simulink model "SPWM_3ph_VSI"  (R2022b)
settings: Solver=FixedStepAuto  StartTime=0.0  StopTime=0.5  RelTol=1e-3
libraries: spsIGBTDiodeLib x6, spsSeriesRLCBranchLib x3, spsDCVoltageSourceLib x2, spsVoltageMeasurementLib x2, spsGroundLib x1, spsTriangleGeneratorLib x1, spspowerguiLib x1
settings Model: Creator=jack  LastModifiedBy=jack

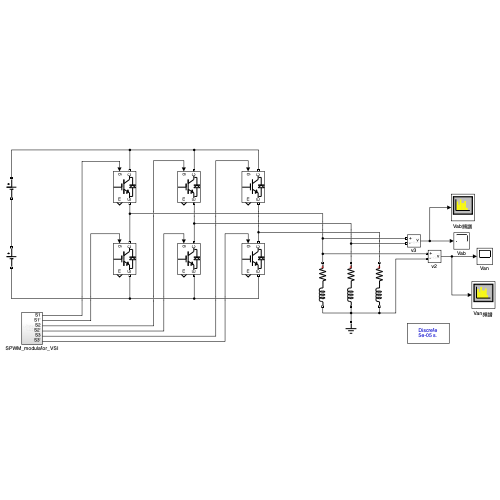
[thumbnail: Simulink's stored preview of the top-level diagram]
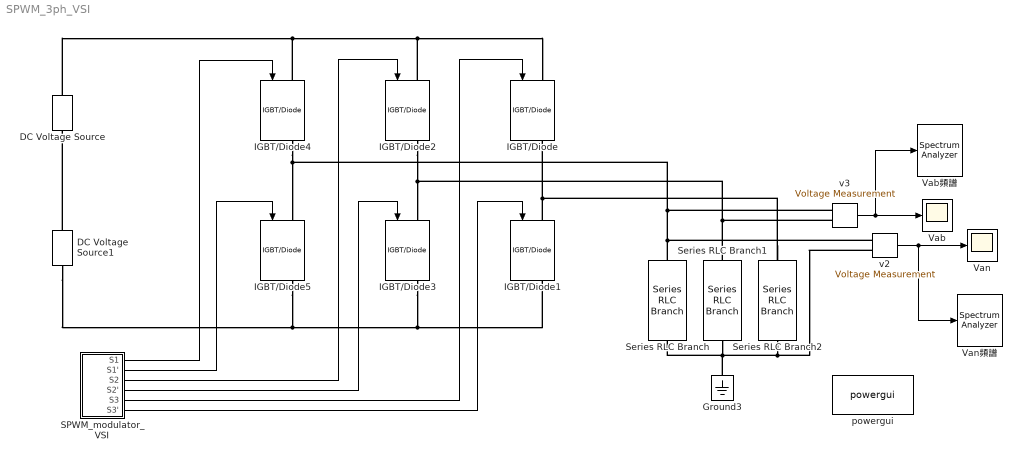
== system SPWM_3ph_VSI ==
  DC Voltage Source : spsDCVoltageSourceLib/DC Voltage Source  Amplitude=100  Measurements=None
  DC Voltage Source1 : spsDCVoltageSourceLib/DC Voltage Source  Amplitude=100  Measurements=None
  Ground3 : spsGroundLib/Ground  LConnTagsString=a
  IGBT/Diode{,1..5} (6 alike) : spsIGBTDiodeLib/IGBT//Diode  Ron=1e-3  Rs=1e5  Cs=inf  Measurements=on
  SPWM_modulator_VSI : Subsystem
  Series RLC Branch : spsSeriesRLCBranchLib/Series RLC Branch  LConnTagsString=__new0  RConnTagsString=__new0  BranchType=RL  Resistance=5  Inductance=150e-3  SetiL0=off  InitialCurrent=0  Capacitance=0  Setx0=off  InitialVoltage=0  Measurements=None
  Series RLC Branch1 : spsSeriesRLCBranchLib/Series RLC Branch  LConnTagsString=__new0  RConnTagsString=__new0  BranchType=RL  Resistance=5  Inductance=150e-3  SetiL0=off  InitialCurrent=0  Capacitance=0  Setx0=off  InitialVoltage=0  Measurements=None
  Series RLC Branch2 : spsSeriesRLCBranchLib/Series RLC Branch  LConnTagsString=__new0  RConnTagsString=__new0  BranchType=RL  Resistance=5  Inductance=150e-3  SetiL0=off  InitialCurrent=0  Capacitance=0  Setx0=off  InitialVoltage=0  Measurements=None
  Vab : Scope
  Vab頻譜 : SpectrumAnalyzer
  Van : Scope
  Van頻譜 : SpectrumAnalyzer
  powergui : spspowerguiLib/powergui  Priority=1  SimulationMode=Discrete  SampleTime=50e-6  frequency=60  Iterations=50  frequencyindice=0  Pbase=100e6  ErrMax=1e-4  UnitsV=kV  UnitsW=MW  buscounter=0  FunctionMessages=off  echomessages=off  EnableUseOfTLC=off  CurrentSourceSwitches=off  DisableSnubberDevices=off  DisableRonSwitches=off  DisableVfSwitches=off  DisplayEquations=off  AutomaticDiscreteSolvers=off  SolverType=Tustin/Backward Euler (TBE)  Interpol=off  ExternalGateDelay=off  methode=off  Ts=100  x0status=blocks  SPID=on  SwTol=0  HookPort=off  NonlinearTolerance=1e-4  nMaxIteration=100  ContinueOnMaxIteration=off  RestoreLinks=warning  ResistiveCurrentMeasurement=off  Frange=[0:2:500]  Ylog=off  Xlog=on  ShowGrid=off  save=off  variable=ZData  structure=0  ZoomFFT=off  StartTime=0.0  cycles=1  DisplayStyle=1  fundamental=60  FreqAxis=off  MaxFrequency=1000  frequencyindicesteady=1  RmsSteady=1  display=off
  v2 : spsVoltageMeasurementLib/Voltage Measurement  PhasorSimulation=off  OutputType=Complex  PSBequivalent=0
  v3 : spsVoltageMeasurementLib/Voltage Measurement  PhasorSimulation=off  OutputType=Complex  PSBequivalent=0
  wires:
  v2/1 -> Van頻譜/1, Van/1
  v3/1 -> Vab頻譜/1, Vab/1
  SPWM_modulator_VSI/1(S1) -> IGBT/Diode4/1
  SPWM_modulator_VSI/2(S1') -> IGBT/Diode5/1
  SPWM_modulator_VSI/3(S2) -> IGBT/Diode2/1
  SPWM_modulator_VSI/4(S2') -> IGBT/Diode3/1
  SPWM_modulator_VSI/5(S3) -> IGBT/Diode/1
  SPWM_modulator_VSI/6(S3') -> IGBT/Diode1/1
  connections:
  IGBT/Diode1/LConn1 -- IGBT/Diode/RConn1 -- Series RLC Branch2/LConn1
  IGBT/Diode1/RConn1 -- DC Voltage Source1/LConn1 -- IGBT/Diode5/RConn1 -- IGBT/Diode3/RConn1
  DC Voltage Source/RConn1 -- IGBT/Diode4/LConn1 -- IGBT/Diode2/LConn1 -- IGBT/Diode/LConn1
  IGBT/Diode2/RConn1 -- Series RLC Branch1/LConn1 -- v3/LConn2 -- IGBT/Diode3/LConn1
  IGBT/Diode4/RConn1 -- v3/LConn1 -- v2/LConn1 -- Series RLC Branch/LConn1 -- IGBT/Diode5/LConn1
  DC Voltage Source1/RConn1 -- DC Voltage Source/LConn1
  Series RLC Branch1/RConn1 -- v2/LConn2 -- Series RLC Branch2/RConn1 -- Series RLC Branch/RConn1 -- Ground3/LConn1

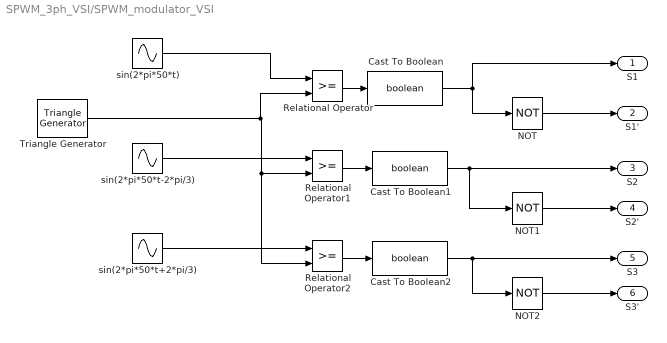
== system SPWM_3ph_VSI/SPWM_modulator_VSI ==
  Cast To Boolean : DataTypeConversion  OutDataTypeStr=boolean  SaturateOnIntegerOverflow=off  RndMeth=Floor
  Cast To Boolean1 : DataTypeConversion  OutDataTypeStr=boolean  SaturateOnIntegerOverflow=off  RndMeth=Floor
  Cast To Boolean2 : DataTypeConversion  OutDataTypeStr=boolean  SaturateOnIntegerOverflow=off  RndMeth=Floor
  NOT : Logic  Operator=NOT  IconShape=distinctive  AllPortsSameDT=off  OutDataTypeStr=boolean
  NOT1 : Logic  Operator=NOT  IconShape=distinctive  AllPortsSameDT=off  OutDataTypeStr=boolean
  NOT2 : Logic  Operator=NOT  IconShape=distinctive  AllPortsSameDT=off  OutDataTypeStr=boolean
  Relational Operator : RelationalOperator  OutDataTypeStr=boolean  RndMeth=Simplest  InputSameDT=off
  Relational Operator1 : RelationalOperator  OutDataTypeStr=boolean  RndMeth=Simplest  InputSameDT=off
  Relational Operator2 : RelationalOperator  OutDataTypeStr=boolean  RndMeth=Simplest  InputSameDT=off
  Triangle Generator : spsTriangleGeneratorLib/Triangle Generator  Freq=2e3  Phase=90  Ts=0
  sin(2*pi*50*t) : Sin  Frequency=2*pi*50  SampleTime=0
  sin(2*pi*50*t+2*pi/3) : Sin  Frequency=2*pi*50  Phase=2*pi/3  SampleTime=0
  sin(2*pi*50*t-2*pi/3) : Sin  Frequency=2*pi*50  Phase=-2*pi/3  SampleTime=0
  S1 : Outport
  S1' : Outport  Port=2
  S2 : Outport  Port=3
  S2' : Outport  Port=4
  S3 : Outport  Port=5
  S3' : Outport  Port=6
  wires:
  NOT/1 -> S1'/1
  Relational Operator/1 -> Cast To Boolean/1
  Cast To Boolean/1 -> S1/1, NOT/1
  Triangle Generator/1 -> Relational Operator/2, Relational Operator2/2, Relational Operator1/2
  sin(2*pi*50*t)/1 -> Relational Operator/1
  Relational Operator1/1 -> Cast To Boolean1/1
  Cast To Boolean1/1 -> S2/1, NOT1/1
  NOT1/1 -> S2'/1
  sin(2*pi*50*t-2*pi/3)/1 -> Relational Operator1/1
  Relational Operator2/1 -> Cast To Boolean2/1
  sin(2*pi*50*t+2*pi/3)/1 -> Relational Operator2/1
  NOT2/1 -> S3'/1
  Cast To Boolean2/1 -> NOT2/1, S3/1
